simulink model "CC_CV_CHARGING"  (R2025a)
settings: Solver=VariableStepAuto  StartTime=0.0  StopTime=200  RelTol=1e-3
undefined symbols (not defined in the file): Ion, Lithium
libraries: spsMosfetLib x2, spsSeriesRLCBranchLib x2, spsBatteryLib x1, spsControlledCurrentSourceLib x1, spsDCVoltageSourceLib x1, spsDiodeLib x1, sps_lib x1
settings Model: Creator=USER  LastModifiedBy=ashis

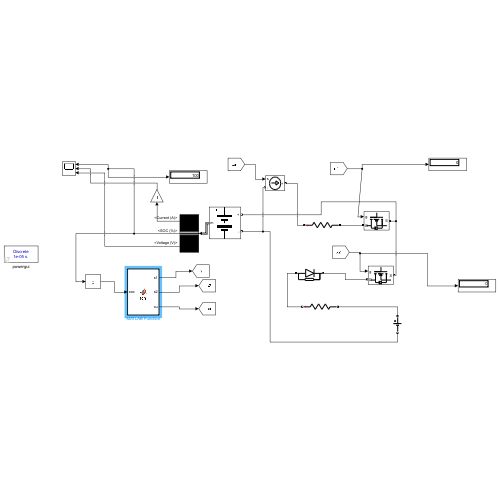
[thumbnail: Simulink's stored preview of the top-level diagram]
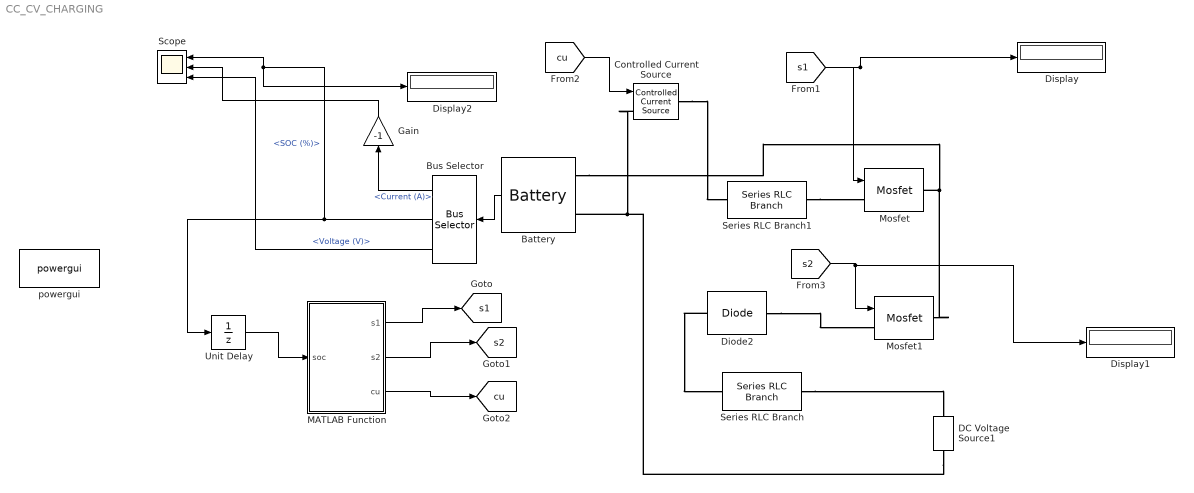
== system CC_CV_CHARGING ==
  Battery : spsBatteryLib/Battery  BatType=Lithium-Ion  NomV=3.3  NomQ=1  SOC=77  Batt_Tr=30  PresetModel=on  MaxQ=1  MinV=2.475  FullV=3.8412  Dis_rate=0.43478  R=0.033  Normal_OP=0.90435  expZone="[3.5653     0.04913]"
  Bus Selector : BusSelector  OutputSignals=Current (A),SOC (%),Voltage (V)
  Controlled Current Source : spsControlledCurrentSourceLib/Controlled Current Source  Initialize=on  Source_Type=DC  Amplitude=10  Phase=0  Frequency=0  Measurements=None
  DC Voltage Source1 : spsDCVoltageSourceLib/DC Voltage Source  Amplitude=3.8  Measurements=None
  Diode2 : spsDiodeLib/Diode  Ron=0.001  Lon=0  Vf=0.8  IC=0  UseSnubber=0  Rs=500  Cs=250e-9  Measurements=off
  Display : Display
  Display1 : Display
  Display2 : Display
  Gain : Gain  Gain=-1
  MATLAB Function : MATLAB Function  TreatAsAtomicUnit=on
  Mosfet : spsMosfetLib/Mosfet  Ron=0.1  Lon=0  Rd=0.01  Vfd=0  IC=0  Rs=1e5  Cs=inf  Measurements=off
  Mosfet1 : spsMosfetLib/Mosfet  Ron=0.1  Lon=0  Rd=0.01  Vfd=0  IC=0  Rs=1e5  Cs=inf  Measurements=off
  Scope : Scope  NumInputPorts=3
      settings: ActiveDisplayYMinimum=74.975822050290077  ActiveDisplayYMaximum=102.78046421663444
  Series RLC Branch : spsSeriesRLCBranchLib/Series RLC Branch  LConnTagsString=__new0  RConnTagsString=__new0  BranchType=R  Resistance=1  Inductance=1e-3  SetiL0=off  InitialCurrent=0  Capacitance=1e-6  Setx0=off  InitialVoltage=0  Measurements=None
  Series RLC Branch1 : spsSeriesRLCBranchLib/Series RLC Branch  LConnTagsString=__new0  RConnTagsString=__new0  BranchType=R  Resistance=0.1  Inductance=1e-3  SetiL0=off  InitialCurrent=0  Capacitance=1e-6  Setx0=off  InitialVoltage=0  Measurements=None
  Unit Delay : UnitDelay  SampleTime=1e-5  HasFrameUpgradeWarning=on
  powergui : sps_lib/powergui  Priority=1  SimulationMode=Discrete  SampleTime=1e-5  frequency=60  Iterations=50  frequencyindice=0  Pbase=100e6  ErrMax=1e-4  UnitsV=kV  UnitsW=MW  buscounter=0  FunctionMessages=off  echomessages=off  EnableUseOfTLC=off  CurrentSourceSwitches=off  DisableSnubberDevices=off  DisableRonSwitches=off  DisableVfSwitches=off  DisplayEquations=off  AutomaticDiscreteSolvers=off  SolverType=Tustin/Backward Euler (TBE)  Interpol=off  ExternalGateDelay=off  methode=off  Ts=100  x0status=blocks  SPID=on  SwTol=0  HookPort=off  NonlinearTolerance=1e-4  nMaxIteration=100  ContinueOnMaxIteration=off  RestoreLinks=warning  ResistiveCurrentMeasurement=off  Frange=[0:2:500]  Ylog=off  Xlog=on  ShowGrid=off  save=off  variable=ZData  structure=0  ZoomFFT=off  StartTime=0.0  cycles=1  DisplayStyle=1  fundamental=60  FreqAxis=off  MaxFrequency=1000  frequencyindicesteady=1  RmsSteady=1  display=off
  tag scope: cu=global, s1=global, s2=global
  wires:
  Battery/1 -> Bus Selector/1
  Bus Selector/2 -> Unit Delay/1, Scope/1, Display2/1  "<SOC (%)>"
  Bus Selector/1 -> Gain/1  "<Current (A)>"
  Bus Selector/3 -> Scope/3  "<Voltage (V)>"
  MATLAB Function/1(s1) -> [s1]
  MATLAB Function/2(s2) -> [s2]
  MATLAB Function/3(cu) -> [cu]
  [cu] -> Controlled Current Source/1
  [s1] -> Mosfet/1, Display/1
  [s2] -> Display1/1, Mosfet1/1
  Unit Delay/1 -> MATLAB Function/1(soc)
  Gain/1 -> Scope/2
  connections:
  Series RLC Branch/RConn1 -- DC Voltage Source1/RConn1
  DC Voltage Source1/LConn1 -- Controlled Current Source/LConn1 -- Battery/LConn2
  Diode2/LConn1 -- Series RLC Branch/LConn1
  Diode2/RConn1 -- Mosfet1/LConn1
  Controlled Current Source/RConn1 -- Series RLC Branch1/LConn1
  Battery/LConn1 -- Mosfet1/RConn1 -- Mosfet/RConn1
  Series RLC Branch1/RConn1 -- Mosfet/LConn1

== matlab function CC_CV_CHARGING/MATLAB Function ==
  data: soc input; s1 output; s2 output; cu output
function [s1,s2,cu] = fcn(soc)

s1 = 0;
s2 = 0;
cu = 0;

% ---------- CC MODE ----------
if ((soc >= 0) && (soc <= 80))

    s1 = 1;
    s2 = 0;
    cu = 10;

% ---------- CV MODE ----------
elseif ((soc > 80) && (soc < 100))

    s1 = 0;
    s2 = 1;
    cu = 4;

% ---------- FULL CHARGE ----------
else

    s1 = 0;
    s2 = 0;
    cu = 0;

end
